simulink model "OscillatorAndLockin_DynamicFreqMod"  (R2022b)
settings: Solver=VariableStepAuto  StartTime=0.0  StopTime=0.6  RelTol=1e-3
model workspace: external: MAT-File C:\Users\yoni\Documents\MATLAB\Examples\AFM\Dynamic Mode\WorkSpaceData.mat (data not in the file)
undefined symbols (not defined in the file or in its folder): ClockPeriod, D, I, N, P
libraries: simulink x7, slpidlib x3, simulink_extras x1
(part 2 of 2)

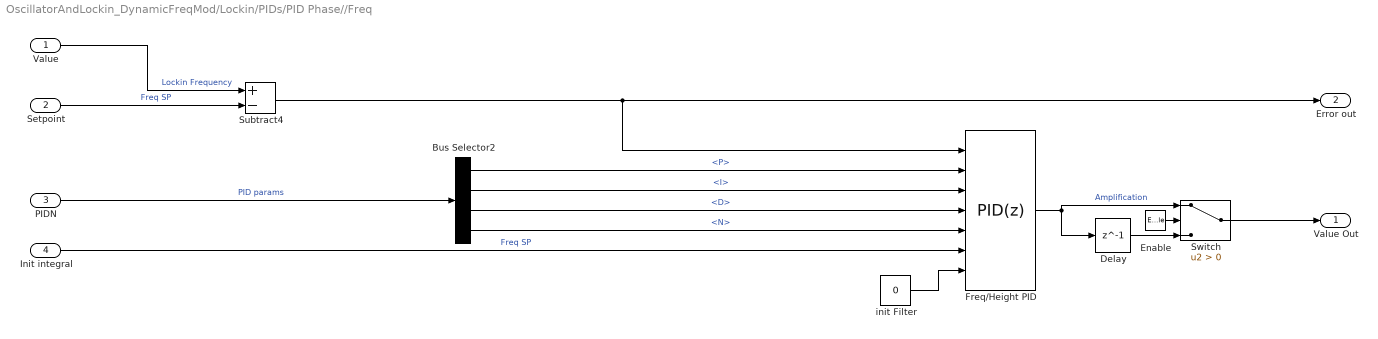
== system OscillatorAndLockin_DynamicFreqMod/Lockin/PIDs/PID Phase//Freq ==
  Value : Inport
  Setpoint : Inport  Port=2
  PIDN : Inport  Port=3
  Init integral : Inport  Port=4
  Enable : EnablePort  ShowOutputPort=on
  Bus Selector2 : BusSelector  OutputSignals=P,I,D,N
  Delay : Delay  DelayLength=1  InitialCondition=0
  Freq/Height PID : slpidlib/PID Controller  Controller=PID  Form=Parallel  TimeDomain=Discrete-time  UseExternalTs=off  SampleTime=-1  IntegratorMethod=Forward Euler  FilterMethod=Forward Euler  ControllerParametersSource=external  P=20  I=100  UseKiTs=off  D=1400  N=1  UseFilter=on  TunerSelectOption=Transfer Function Based (PID Tuner App)  InitialConditionSource=external  InitialConditionForIntegrator=0  InitialConditionForFilter=0  DifferentiatorICPrevScaledInput=0  ExternalReset=none  TrackingMode=off  Kt=1  LimitOutput=off  SatLimitsSource=internal  UpperSaturationLimit=inf  LowerSaturationLimit=-inf  LinearizeAsGain=off  AntiWindupMode=none  Kb=1  LimitIntegrator=off  UpperIntegratorSaturationLimit=inf  LowerIntegratorSaturationLimit=-inf  RndMeth=Round  POutMin=[]  POutMax=[]  IOutMin=[]  IOutMax=[]  DOutMin=[]  DOutMax=[]  NOutMin=[]  NOutMax=[]  SumOutMin=[]  SumOutMax=[]  SaturationOutMin=[]  SaturationOutMax=[]  PParamMin=[]  PParamMax=[]  IParamMin=[]  IParamMax=[]  DParamMin=[]  DParamMax=[]  NParamMin=[]  NParamMax=[]  KbParamMin=[]  KbParamMax=[]  KtParamMin=[]  KtParamMax=[]  KbOutMin=[]  KbOutMax=[]  KtOutMin=[]  KtOutMax=[]  IntegratorOutMin=[]  IntegratorOutMax=[]  FilterOutMin=[]  FilterOutMax=[]  SumI1OutMin=[]  SumI1OutMax=[]  SumI2OutMin=[]  SumI2OutMax=[]  SumI3OutMin=[]  SumI3OutMax=[]  SumI4OutMin=[]  SumI4OutMax=[]  SumDOutMin=[]  SumDOutMax=[]  DifferentiatorOutMin=[]  DifferentiatorOutMax=[]  FilterDiffOutCoefMin=[]  FilterDiffOutCoefMax=[]  ReciprocalOutMin=[]  ReciprocalOutMax=[]  SumDenOutMin=[]  SumDenOutMax=[]  SumNumOutMin=[]  SumNumOutMax=[]  DivideOutMin=[]  DivideOutMax=[]  UdiffTsProdOutMin=[]  UdiffTsProdOutMax=[]  NTsProdOutMin=[]  NTsProdOutMax=[]  UintegralTsProdOutMin=[]  UintegralTsProdOutMax=[]  UngainTsProdOutMin=[]  UngainTsProdOutMax=[]  ClampingZeroOutDataTypeStr=Inherit: Inherit via back propagation  ClampingZeroOutMin=[]  ClampingZeroOutMax=[]  FilterDenConstantOutDataTypeStr=Inherit: Inherit via back propagation  FilterDenConstantOutMin=[]  FilterDenConstantOutMax=[]  PCopyOutDataTypeStr=Inherit: Inherit via back propagation  PCopyOutMin=[]  PCopyOutMax=[]  NCopyOutDataTypeStr=Inherit: Inherit via back propagation  NCopyOutMin=[]  NCopyOutMax=[]  IntegratorContinuousStateAttributes=''  IntegratorStateMustResolveToSignalObject=off  IntegratorRTWStateStorageClass=Auto  FilterContinuousStateAttributes=''  FilterStateMustResolveToSignalObject=off  FilterRTWStateStorageClass=Auto  ParallelPVariant=ExternalParameters  IdealPVariant=Disabled  IVariant=ExternalParameters  DVariant=ExternalParameters  IntegratorVariant=Discrete  SatVariant=Disabled  AWVariant=Passthrough  PCopyVariant=Disabled  TRVariant=Disabled  FdbkBlocksVariant=Forward  IdealPFdbkVariant=Disabled  SatFdbkVariant=Disabled  DerivativeFilterVariant=ForwardEulerFilter  NVariant=ExternalParameters  NCopyVariant=Disabled  FilterICVariant=ExternalICs  IntegratorICVariant=ExternalICs  ExternalResetVariant=Disabled  TRSumVariant=Passthrough  SumFdbkVariant=Disabled  SumVariant=Sum_PID  TsampFilterVariant=InternalTs  TsampNgainVariant=Passthrough  TsampIntegralVariant=Passthrough  ExternalSaturationOutDataTypeStr=Inherit: Same as second input
  Subtract4 : Sum  Inputs=+-
  Switch : Switch  Criteria=u2 > Threshold  SaturateOnIntegerOverflow=off  InputSameDT=off
  init Filter : Constant  Value=0
  Value Out : Outport
  Error out : Outport  Port=2
  wires:
  Subtract4/1 -> Freq/Height PID/1, Error out/1
  Setpoint/1 -> Subtract4/2  "Freq SP"
  Bus Selector2/2 -> Freq/Height PID/3  "<I>"
  Bus Selector2/3 -> Freq/Height PID/4  "<D>"
  PIDN/1 -> Bus Selector2/1  "PID params"
  Value/1 -> Subtract4/1  "Lockin Frequency"
  Bus Selector2/4 -> Freq/Height PID/5  "<N>"
  Bus Selector2/1 -> Freq/Height PID/2  "<P>"
  Freq/Height PID/1 -> Switch/1, Delay/1  "Amplification"
  Delay/1 -> Switch/3
  Enable/1 -> Switch/2
  Switch/1 -> Value Out/1
  Init integral/1 -> Freq/Height PID/6  "Freq SP"
  init Filter/1 -> Freq/Height PID/7

== matlab function OscillatorAndLockin_DynamicFreqMod/MATLAB Function1 ==
  data: SeparationDistance input; Force output; Potential output
%% Calculates the interaction Force and Potential as a function of seperation distance
function [Force,Potential] = TipSampleInteraction(SeparationDistance)
[Potential,Force] = sampledistanceLJ(SeparationDistance);
